simulink model "Sim2g"  (R2016a)
settings: Solver=VariableStepAuto  StartTime=0.0  StopTime=total_time  RelTol=1e-3
values from neighbouring files (symbols this model uses):
  A = [-0.322 0.052 0.028 -1.12   0.002 ... (first row only)    [modelParms.m]
  antiWindupBound = 0.3    [modelParms.m]
  B = [0 0 0 0 10]'    [modelParms.m]
  dist = deg2rad(2)    [modelParms.m]
  g = 9.8    [modelParms.m]
  k_d_phi = (2*zeta_phi*omega_n_phi - alpha_phi1)/alpha_phi2    [modelParms.m]
  k_i_chi = omega_n_chi^2*V_g/g    [AllResults.m]    (also in modelParms.m)
  k_p_chi = 2*zeta_chi*omega_n_chi*V_g/g    [AllResults.m]    (also in modelParms.m)
  k_p_phi = delta_a_max/e_phi_max * sign(alpha_phi2)    [modelParms.m]
  V_g = 637    [modelParms.m]
settings Model: Creator=Alex  LastModifiedBy=Alex

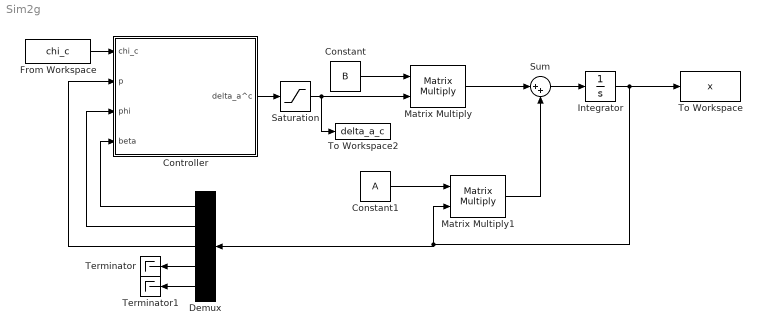
== system Sim2g ==
  Constant : Constant  Value=B
  Constant1 : Constant  Value=A
  Controller : Subsystem
  Demux : Demux  Outputs=5
  From Workspace : FromWorkspace  VariableName=chi_c  SampleTime=0
  Integrator : Integrator
  Matrix Multiply : Product  Multiplication=Matrix(*)
  Matrix Multiply1 : Product  Multiplication=Matrix(*)
  Saturation : Saturate  UpperLimit=deg2rad(25)  LowerLimit=deg2rad(-25)
  Sum : Sum  Inputs=|++
  Terminator : Terminator
  Terminator1 : Terminator
  To Workspace : ToWorkspace  VariableName=x  SaveFormat=Timeseries  SampleTime=-1
  To Workspace2 : ToWorkspace  VariableName=delta_a_c  SaveFormat=Timeseries  SampleTime=-1
  wires:
  Controller/1(delta_a^c) -> Saturation/1
  Constant/1 -> Matrix Multiply/1
  Matrix Multiply/1 -> Sum/1
  Matrix Multiply1/1 -> Sum/2
  Constant1/1 -> Matrix Multiply1/1
  Sum/1 -> Integrator/1
  Demux/1 -> Controller/4(beta)
  Demux/2 -> Controller/3(phi)
  Demux/4 -> Terminator/1
  Demux/5 -> Terminator1/1
  Saturation/1 -> To Workspace2/1, Matrix Multiply/2
  Demux/3 -> Controller/2(p)
  From Workspace/1 -> Controller/1(chi_c)
  Integrator/1 -> Matrix Multiply1/2, Demux/1, To Workspace/1

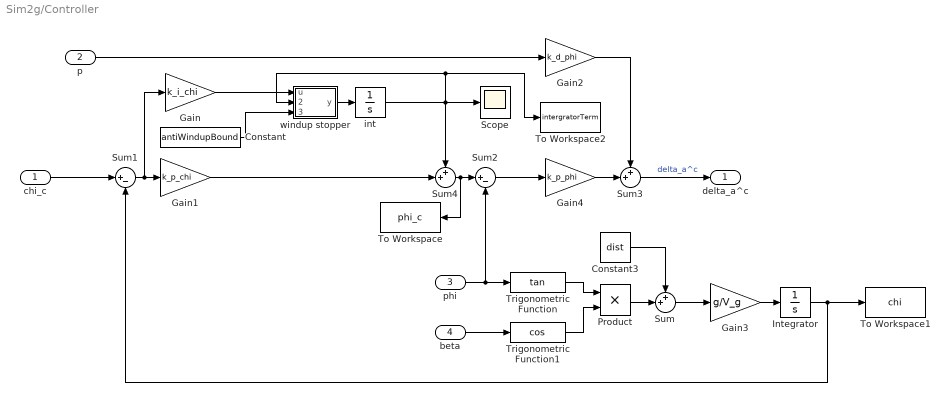
== system Sim2g/Controller ==
  chi_c : Inport
  p : Inport  Port=2
  phi : Inport  Port=3
  beta : Inport  Port=4
  Constant : Constant  Value=antiWindupBound
  Constant3 : Constant  Value=dist
  Gain : Gain  Gain=k_i_chi
  Gain1 : Gain  Gain=k_p_chi
  Gain2 : Gain  Gain=k_d_phi
  Gain3 : Gain  Gain=g/V_g
  Gain4 : Gain  Gain=k_p_phi
  Integrator : Integrator
  Product : Product
  Scope : Scope
  Sum : Sum  Inputs=++|
  Sum1 : Sum  Inputs=|+-
  Sum2 : Sum  Inputs=|+-
  Sum3 : Sum  Inputs=++|
  Sum4 : Sum  Inputs=++|
  To Workspace : ToWorkspace  VariableName=phi_c  SaveFormat=Timeseries  SampleTime=-1
  To Workspace1 : ToWorkspace  VariableName=chi  SaveFormat=Timeseries  SampleTime=-1
  To Workspace2 : ToWorkspace  VariableName=intergratorTerm  SaveFormat=Timeseries  SampleTime=-1
  Trigonometric Function : Trigonometry  Operator=tan
  Trigonometric Function1 : Trigonometry  Operator=cos
  int : Integrator
  windup stopper : MATLAB Function  TreatAsAtomicUnit=on
  delta_a^c : Outport
  wires:
  Sum3/1 -> delta_a^c/1  "delta_a^c"
  Gain3/1 -> Integrator/1
  Trigonometric Function1/1 -> Product/2
  Trigonometric Function/1 -> Product/1
  beta/1 -> Trigonometric Function1/1
  Gain4/1 -> Sum3/2
  Sum4/1 -> To Workspace/1, Sum2/1
  p/1 -> Gain2/1
  chi_c/1 -> Sum1/1
  Gain1/1 -> Sum4/2
  Sum1/1 -> Gain1/1, Gain/1
  Sum2/1 -> Gain4/1
  Gain2/1 -> Sum3/1
  int/1 -> Scope/1, windup stopper/2(compare), To Workspace2/1, Sum4/1
  phi/1 -> Sum2/2, Trigonometric Function/1
  Integrator/1 -> Sum1/2, To Workspace1/1
  Gain/1 -> windup stopper/1(u)
  windup stopper/1(y) -> int/1
  Constant/1 -> windup stopper/3(antiWindupBound)
  Product/1 -> Sum/2
  Constant3/1 -> Sum/1
  Sum/1 -> Gain3/1

== matlab function Sim2g/Controller/windup stopper ==
  data: u input; y output; compare input; antiWindupBound input
function y = fcn(u,compare, antiWindupBound)
%#codegen
if((abs(compare) >= antiWindupBound) && sign(u) == sign(compare))
    y = 0;
else
    y=u;
end
